simulink model "VCU_CS75_10_9_SteeringTorque"  (R2014a)
settings: Solver=FixedStepDiscrete  StartTime=0.0  StopTime=25  FixedStep=0.0005  RelTol=1e-3
undefined symbols (not defined in the file or in its folder): AutoDrivingReady, ecucoder_acal, I_SW01_L, LaterlAngleCommand, LDW, RemoteAcclPosition
libraries: simulink x880, ec5744lib x37
(part 19 of 30)

== system VCU_CS75_10_9_SteeringTorque/长安CS75底盘程序，20ms一次/Output/Subsystem/TransmitMessages10/LAS_29D/LAS_LDWShakeLevStatus ==
  LAS_LDWShakeLevStatus : Inport
  Constant{1,3..8} (7 alike) : Constant  Value=0  OutDataTypeStr=uint8
  LAS_LDWShakeLevStatusRon : Rounding  Operator=round
  LAS_LDWShakeLevStatus_1sat : Saturate  UpperLimit=48  LowerLimit=0
  LAS_LDWShakeLevStatus_Convert : DataTypeConversion  OutDataTypeStr=uint8
  LAS_LDWShakeLevStatus_Convert1 : DataTypeConversion  OutDataTypeStr=uint32
  LAS_LDWShakeLevStatus_D : Product  Inputs=*/
  LAS_LDWShakeLevStatus_F : Constant  OutDataTypeStr=single
  LAS_LDWShakeLevStatus_L : simulink/Logic and Bit Operations/Bitwise Operator  logicop=AND  UseBitMask=on  BitMask=48  BitMaskRealWorld=Stored Integer
  LAS_LDWShakeLevStatus_O : Constant  Value=0  OutDataTypeStr=single
  LAS_LDWShakeLevStatus_S : ArithShift  BitShiftNumber=-4
  LAS_LDWShakeLevStatus_sat : Saturate  UpperLimit=3  LowerLimit=0
  LAS_LDWShakeLevStatus_st : Sum  Inputs=+-
  output1 : Outport
  output2 : Outport  Port=2
  output3 : Outport  Port=3
  output4 : Outport  Port=4
  output5 : Outport  Port=5
  output6 : Outport  Port=6
  output7 : Outport  Port=7
  output8 : Outport  Port=8
  wires:
  LAS_LDWShakeLevStatus/1 -> LAS_LDWShakeLevStatus_sat/1
  LAS_LDWShakeLevStatus_sat/1 -> LAS_LDWShakeLevStatus_st/1
  LAS_LDWShakeLevStatus_O/1 -> LAS_LDWShakeLevStatus_st/2
  LAS_LDWShakeLevStatus_st/1 -> LAS_LDWShakeLevStatus_D/1
  LAS_LDWShakeLevStatus_F/1 -> LAS_LDWShakeLevStatus_D/2
  LAS_LDWShakeLevStatus_D/1 -> LAS_LDWShakeLevStatusRon/1
  LAS_LDWShakeLevStatusRon/1 -> LAS_LDWShakeLevStatus_S/1
  LAS_LDWShakeLevStatus_S/1 -> LAS_LDWShakeLevStatus_1sat/1
  LAS_LDWShakeLevStatus_1sat/1 -> LAS_LDWShakeLevStatus_Convert1/1
  LAS_LDWShakeLevStatus_Convert1/1 -> LAS_LDWShakeLevStatus_L/1
  LAS_LDWShakeLevStatus_L/1 -> LAS_LDWShakeLevStatus_Convert/1
  LAS_LDWShakeLevStatus_Convert/1 -> output2/1
  Constant1/1 -> output1/1
  Constant3/1 -> output3/1
  Constant4/1 -> output4/1
  Constant5/1 -> output5/1
  Constant6/1 -> output6/1
  Constant7/1 -> output7/1
  Constant8/1 -> output8/1

== system VCU_CS75_10_9_SteeringTorque/长安CS75底盘程序，20ms一次/Output/Subsystem/TransmitMessages10/LAS_29D/LAS_LLaneMarkerType ==
  LAS_LLaneMarkerType : Inport
  Constant{1..4,6..8} (7 alike) : Constant  Value=0  OutDataTypeStr=uint8
  LAS_LLaneMarkerTypeRon : Rounding  Operator=round
  LAS_LLaneMarkerType_1sat : Saturate  UpperLimit=7  LowerLimit=0
  LAS_LLaneMarkerType_Convert : DataTypeConversion  OutDataTypeStr=uint8
  LAS_LLaneMarkerType_Convert1 : DataTypeConversion  OutDataTypeStr=uint32
  LAS_LLaneMarkerType_D : Product  Inputs=*/
  LAS_LLaneMarkerType_F : Constant  OutDataTypeStr=single
  LAS_LLaneMarkerType_L : simulink/Logic and Bit Operations/Bitwise Operator  logicop=AND  UseBitMask=on  BitMask=7  BitMaskRealWorld=Stored Integer
  LAS_LLaneMarkerType_O : Constant  Value=0  OutDataTypeStr=single
  LAS_LLaneMarkerType_S : ArithShift
  LAS_LLaneMarkerType_sat : Saturate  UpperLimit=7  LowerLimit=0
  LAS_LLaneMarkerType_st : Sum  Inputs=+-
  output1 : Outport
  output2 : Outport  Port=2
  output3 : Outport  Port=3
  output4 : Outport  Port=4
  output5 : Outport  Port=5
  output6 : Outport  Port=6
  output7 : Outport  Port=7
  output8 : Outport  Port=8
  wires:
  LAS_LLaneMarkerType/1 -> LAS_LLaneMarkerType_sat/1
  LAS_LLaneMarkerType_sat/1 -> LAS_LLaneMarkerType_st/1
  LAS_LLaneMarkerType_O/1 -> LAS_LLaneMarkerType_st/2
  LAS_LLaneMarkerType_st/1 -> LAS_LLaneMarkerType_D/1
  LAS_LLaneMarkerType_F/1 -> LAS_LLaneMarkerType_D/2
  LAS_LLaneMarkerType_D/1 -> LAS_LLaneMarkerTypeRon/1
  LAS_LLaneMarkerTypeRon/1 -> LAS_LLaneMarkerType_S/1
  LAS_LLaneMarkerType_S/1 -> LAS_LLaneMarkerType_1sat/1
  LAS_LLaneMarkerType_1sat/1 -> LAS_LLaneMarkerType_Convert1/1
  LAS_LLaneMarkerType_Convert1/1 -> LAS_LLaneMarkerType_L/1
  LAS_LLaneMarkerType_L/1 -> LAS_LLaneMarkerType_Convert/1
  LAS_LLaneMarkerType_Convert/1 -> output5/1
  Constant1/1 -> output1/1
  Constant2/1 -> output2/1
  Constant3/1 -> output3/1
  Constant4/1 -> output4/1
  Constant6/1 -> output6/1
  Constant7/1 -> output7/1
  Constant8/1 -> output8/1

== system VCU_CS75_10_9_SteeringTorque/长安CS75底盘程序，20ms一次/Output/Subsystem/TransmitMessages10/LAS_29D/LAS_LdwSensitivityStatus ==
  LAS_LdwSensitivityStatus : Inport
  Constant{2..8} (7 alike) : Constant  Value=0  OutDataTypeStr=uint8
  LAS_LdwSensitivityStatusRon : Rounding  Operator=round
  LAS_LdwSensitivityStatus_1sat : Saturate  UpperLimit=192  LowerLimit=0
  LAS_LdwSensitivityStatus_Convert : DataTypeConversion  OutDataTypeStr=uint8
  LAS_LdwSensitivityStatus_Convert1 : DataTypeConversion  OutDataTypeStr=uint32
  LAS_LdwSensitivityStatus_D : Product  Inputs=*/
  LAS_LdwSensitivityStatus_F : Constant  OutDataTypeStr=single
  LAS_LdwSensitivityStatus_L : simulink/Logic and Bit Operations/Bitwise Operator  logicop=AND  UseBitMask=on  BitMask=192  BitMaskRealWorld=Stored Integer
  LAS_LdwSensitivityStatus_O : Constant  Value=0  OutDataTypeStr=single
  LAS_LdwSensitivityStatus_S : ArithShift  BitShiftNumber=-6
  LAS_LdwSensitivityStatus_sat : Saturate  UpperLimit=3  LowerLimit=0
  LAS_LdwSensitivityStatus_st : Sum  Inputs=+-
  output1 : Outport
  output2 : Outport  Port=2
  output3 : Outport  Port=3
  output4 : Outport  Port=4
  output5 : Outport  Port=5
  output6 : Outport  Port=6
  output7 : Outport  Port=7
  output8 : Outport  Port=8
  wires:
  LAS_LdwSensitivityStatus/1 -> LAS_LdwSensitivityStatus_sat/1
  LAS_LdwSensitivityStatus_sat/1 -> LAS_LdwSensitivityStatus_st/1
  LAS_LdwSensitivityStatus_O/1 -> LAS_LdwSensitivityStatus_st/2
  LAS_LdwSensitivityStatus_st/1 -> LAS_LdwSensitivityStatus_D/1
  LAS_LdwSensitivityStatus_F/1 -> LAS_LdwSensitivityStatus_D/2
  LAS_LdwSensitivityStatus_D/1 -> LAS_LdwSensitivityStatusRon/1
  LAS_LdwSensitivityStatusRon/1 -> LAS_LdwSensitivityStatus_S/1
  LAS_LdwSensitivityStatus_S/1 -> LAS_LdwSensitivityStatus_1sat/1
  LAS_LdwSensitivityStatus_1sat/1 -> LAS_LdwSensitivityStatus_Convert1/1
  LAS_LdwSensitivityStatus_Convert1/1 -> LAS_LdwSensitivityStatus_L/1
  LAS_LdwSensitivityStatus_L/1 -> LAS_LdwSensitivityStatus_Convert/1
  LAS_LdwSensitivityStatus_Convert/1 -> output1/1
  Constant2/1 -> output2/1
  Constant3/1 -> output3/1
  Constant4/1 -> output4/1
  Constant5/1 -> output5/1
  Constant6/1 -> output6/1
  Constant7/1 -> output7/1
  Constant8/1 -> output8/1

== system VCU_CS75_10_9_SteeringTorque/长安CS75底盘程序，20ms一次/Output/Subsystem/TransmitMessages10/LAS_29D/LAS_OverspeedSoundWarning ==
  LAS_OverspeedSoundWarning : Inport
  Constant{1..3,5..8} (7 alike) : Constant  Value=0  OutDataTypeStr=uint8
  LAS_OverspeedSoundWarningRon : Rounding  Operator=round
  LAS_OverspeedSoundWarning_1sat : Saturate  UpperLimit=192  LowerLimit=0
  LAS_OverspeedSoundWarning_Convert : DataTypeConversion  OutDataTypeStr=uint8
  LAS_OverspeedSoundWarning_Convert1 : DataTypeConversion  OutDataTypeStr=uint32
  LAS_OverspeedSoundWarning_D : Product  Inputs=*/
  LAS_OverspeedSoundWarning_F : Constant  OutDataTypeStr=single
  LAS_OverspeedSoundWarning_L : simulink/Logic and Bit Operations/Bitwise Operator  logicop=AND  UseBitMask=on  BitMask=192  BitMaskRealWorld=Stored Integer
  LAS_OverspeedSoundWarning_O : Constant  Value=0  OutDataTypeStr=single
  LAS_OverspeedSoundWarning_S : ArithShift  BitShiftNumber=-6
  LAS_OverspeedSoundWarning_sat : Saturate  UpperLimit=3  LowerLimit=0
  LAS_OverspeedSoundWarning_st : Sum  Inputs=+-
  output1 : Outport
  output2 : Outport  Port=2
  output3 : Outport  Port=3
  output4 : Outport  Port=4
  output5 : Outport  Port=5
  output6 : Outport  Port=6
  output7 : Outport  Port=7
  output8 : Outport  Port=8
  wires:
  LAS_OverspeedSoundWarning/1 -> LAS_OverspeedSoundWarning_sat/1
  LAS_OverspeedSoundWarning_sat/1 -> LAS_OverspeedSoundWarning_st/1
  LAS_OverspeedSoundWarning_O/1 -> LAS_OverspeedSoundWarning_st/2
  LAS_OverspeedSoundWarning_st/1 -> LAS_OverspeedSoundWarning_D/1
  LAS_OverspeedSoundWarning_F/1 -> LAS_OverspeedSoundWarning_D/2
  LAS_OverspeedSoundWarning_D/1 -> LAS_OverspeedSoundWarningRon/1
  LAS_OverspeedSoundWarningRon/1 -> LAS_OverspeedSoundWarning_S/1
  LAS_OverspeedSoundWarning_S/1 -> LAS_OverspeedSoundWarning_1sat/1
  LAS_OverspeedSoundWarning_1sat/1 -> LAS_OverspeedSoundWarning_Convert1/1
  LAS_OverspeedSoundWarning_Convert1/1 -> LAS_OverspeedSoundWarning_L/1
  LAS_OverspeedSoundWarning_L/1 -> LAS_OverspeedSoundWarning_Convert/1
  LAS_OverspeedSoundWarning_Convert/1 -> output4/1
  Constant1/1 -> output1/1
  Constant2/1 -> output2/1
  Constant3/1 -> output3/1
  Constant5/1 -> output5/1
  Constant6/1 -> output6/1
  Constant7/1 -> output7/1
  Constant8/1 -> output8/1

== system VCU_CS75_10_9_SteeringTorque/长安CS75底盘程序，20ms一次/Output/Subsystem/TransmitMessages10/LAS_29D/LAS_OverspeedSoundWarningEnSt ==
  LAS_OverspeedSoundWarningEnSt : Inport
  Constant{1,3..8} (7 alike) : Constant  Value=0  OutDataTypeStr=uint8
  LAS_OverspeedSoundWarningEnStRon : Rounding  Operator=round
  LAS_OverspeedSoundWarningEnSt_1sat : Saturate  UpperLimit=3  LowerLimit=0
  LAS_OverspeedSoundWarningEnSt_Convert : DataTypeConversion  OutDataTypeStr=uint8
  LAS_OverspeedSoundWarningEnSt_Convert1 : DataTypeConversion  OutDataTypeStr=uint32
  LAS_OverspeedSoundWarningEnSt_D : Product  Inputs=*/
  LAS_OverspeedSoundWarningEnSt_F : Constant  OutDataTypeStr=single
  LAS_OverspeedSoundWarningEnSt_L : simulink/Logic and Bit Operations/Bitwise Operator  logicop=AND  UseBitMask=on  BitMask=3  BitMaskRealWorld=Stored Integer
  LAS_OverspeedSoundWarningEnSt_O : Constant  Value=0  OutDataTypeStr=single
  LAS_OverspeedSoundWarningEnSt_S : ArithShift
  LAS_OverspeedSoundWarningEnSt_sat : Saturate  UpperLimit=3  LowerLimit=0
  LAS_OverspeedSoundWarningEnSt_st : Sum  Inputs=+-
  output1 : Outport
  output2 : Outport  Port=2
  output3 : Outport  Port=3
  output4 : Outport  Port=4
  output5 : Outport  Port=5
  output6 : Outport  Port=6
  output7 : Outport  Port=7
  output8 : Outport  Port=8
  wires:
  LAS_OverspeedSoundWarningEnSt/1 -> LAS_OverspeedSoundWarningEnSt_sat/1
  LAS_OverspeedSoundWarningEnSt_sat/1 -> LAS_OverspeedSoundWarningEnSt_st/1
  LAS_OverspeedSoundWarningEnSt_O/1 -> LAS_OverspeedSoundWarningEnSt_st/2
  LAS_OverspeedSoundWarningEnSt_st/1 -> LAS_OverspeedSoundWarningEnSt_D/1
  LAS_OverspeedSoundWarningEnSt_F/1 -> LAS_OverspeedSoundWarningEnSt_D/2
  LAS_OverspeedSoundWarningEnSt_D/1 -> LAS_OverspeedSoundWarningEnStRon/1
  LAS_OverspeedSoundWarningEnStRon/1 -> LAS_OverspeedSoundWarningEnSt_S/1
  LAS_OverspeedSoundWarningEnSt_S/1 -> LAS_OverspeedSoundWarningEnSt_1sat/1
  LAS_OverspeedSoundWarningEnSt_1sat/1 -> LAS_OverspeedSoundWarningEnSt_Convert1/1
  LAS_OverspeedSoundWarningEnSt_Convert1/1 -> LAS_OverspeedSoundWarningEnSt_L/1
  LAS_OverspeedSoundWarningEnSt_L/1 -> LAS_OverspeedSoundWarningEnSt_Convert/1
  LAS_OverspeedSoundWarningEnSt_Convert/1 -> output2/1
  Constant1/1 -> output1/1
  Constant3/1 -> output3/1
  Constant4/1 -> output4/1
  Constant5/1 -> output5/1
  Constant6/1 -> output6/1
  Constant7/1 -> output7/1
  Constant8/1 -> output8/1

== system VCU_CS75_10_9_SteeringTorque/长安CS75底盘程序，20ms一次/Output/Subsystem/TransmitMessages10/LAS_29D/LAS_OverspeedVisualWarning ==
  LAS_OverspeedVisualWarning : Inport
  Constant{1..4,6..8} (7 alike) : Constant  Value=0  OutDataTypeStr=uint8
  LAS_OverspeedVisualWarningRon : Rounding  Operator=round
  LAS_OverspeedVisualWarning_1sat : Saturate  UpperLimit=192  LowerLimit=0
  LAS_OverspeedVisualWarning_Convert : DataTypeConversion  OutDataTypeStr=uint8
  LAS_OverspeedVisualWarning_Convert1 : DataTypeConversion  OutDataTypeStr=uint32
  LAS_OverspeedVisualWarning_D : Product  Inputs=*/
  LAS_OverspeedVisualWarning_F : Constant  OutDataTypeStr=single
  LAS_OverspeedVisualWarning_L : simulink/Logic and Bit Operations/Bitwise Operator  logicop=AND  UseBitMask=on  BitMask=192  BitMaskRealWorld=Stored Integer
  LAS_OverspeedVisualWarning_O : Constant  Value=0  OutDataTypeStr=single
  LAS_OverspeedVisualWarning_S : ArithShift  BitShiftNumber=-6
  LAS_OverspeedVisualWarning_sat : Saturate  UpperLimit=3  LowerLimit=0
  LAS_OverspeedVisualWarning_st : Sum  Inputs=+-
  output1 : Outport
  output2 : Outport  Port=2
  output3 : Outport  Port=3
  output4 : Outport  Port=4
  output5 : Outport  Port=5
  output6 : Outport  Port=6
  output7 : Outport  Port=7
  output8 : Outport  Port=8
  wires:
  LAS_OverspeedVisualWarning/1 -> LAS_OverspeedVisualWarning_sat/1
  LAS_OverspeedVisualWarning_sat/1 -> LAS_OverspeedVisualWarning_st/1
  LAS_OverspeedVisualWarning_O/1 -> LAS_OverspeedVisualWarning_st/2
  LAS_OverspeedVisualWarning_st/1 -> LAS_OverspeedVisualWarning_D/1
  LAS_OverspeedVisualWarning_F/1 -> LAS_OverspeedVisualWarning_D/2
  LAS_OverspeedVisualWarning_D/1 -> LAS_OverspeedVisualWarningRon/1
  LAS_OverspeedVisualWarningRon/1 -> LAS_OverspeedVisualWarning_S/1
  LAS_OverspeedVisualWarning_S/1 -> LAS_OverspeedVisualWarning_1sat/1
  LAS_OverspeedVisualWarning_1sat/1 -> LAS_OverspeedVisualWarning_Convert1/1
  LAS_OverspeedVisualWarning_Convert1/1 -> LAS_OverspeedVisualWarning_L/1
  LAS_OverspeedVisualWarning_L/1 -> LAS_OverspeedVisualWarning_Convert/1
  LAS_OverspeedVisualWarning_Convert/1 -> output5/1
  Constant1/1 -> output1/1
  Constant2/1 -> output2/1
  Constant3/1 -> output3/1
  Constant4/1 -> output4/1
  Constant6/1 -> output6/1
  Constant7/1 -> output7/1
  Constant8/1 -> output8/1

== system VCU_CS75_10_9_SteeringTorque/长安CS75底盘程序，20ms一次/Output/Subsystem/TransmitMessages10/LAS_29D/LAS_OverspeedWarningEnableStatus ==
  LAS_OverspeedWarningEnableStatus : Inport
  Constant{1..3,5..8} (7 alike) : Constant  Value=0  OutDataTypeStr=uint8
  LAS_OverspeedWarningEnableStatusRon : Rounding  Operator=round
  LAS_OverspeedWarningEnableStatus_1sat : Saturate  UpperLimit=48  LowerLimit=0
  LAS_OverspeedWarningEnableStatus_Convert : DataTypeConversion  OutDataTypeStr=uint8
  LAS_OverspeedWarningEnableStatus_Convert1 : DataTypeConversion  OutDataTypeStr=uint32
  LAS_OverspeedWarningEnableStatus_D : Product  Inputs=*/
  LAS_OverspeedWarningEnableStatus_F : Constant  OutDataTypeStr=single
  LAS_OverspeedWarningEnableStatus_L : simulink/Logic and Bit Operations/Bitwise Operator  logicop=AND  UseBitMask=on  BitMask=48  BitMaskRealWorld=Stored Integer
  LAS_OverspeedWarningEnableStatus_O : Constant  Value=0  OutDataTypeStr=single
  LAS_OverspeedWarningEnableStatus_S : ArithShift  BitShiftNumber=-4
  LAS_OverspeedWarningEnableStatus_sat : Saturate  UpperLimit=3  LowerLimit=0
  LAS_OverspeedWarningEnableStatus_st : Sum  Inputs=+-
  output1 : Outport
  output2 : Outport  Port=2
  output3 : Outport  Port=3
  output4 : Outport  Port=4
  output5 : Outport  Port=5
  output6 : Outport  Port=6
  output7 : Outport  Port=7
  output8 : Outport  Port=8
  wires:
  LAS_OverspeedWarningEnableStatus/1 -> LAS_OverspeedWarningEnableStatus_sat/1
  LAS_OverspeedWarningEnableStatus_sat/1 -> LAS_OverspeedWarningEnableStatus_st/1
  LAS_OverspeedWarningEnableStatus_O/1 -> LAS_OverspeedWarningEnableStatus_st/2
  LAS_OverspeedWarningEnableStatus_st/1 -> LAS_OverspeedWarningEnableStatus_D/1
  LAS_OverspeedWarningEnableStatus_F/1 -> LAS_OverspeedWarningEnableStatus_D/2
  LAS_OverspeedWarningEnableStatus_D/1 -> LAS_OverspeedWarningEnableStatusRon/1
  LAS_OverspeedWarningEnableStatusRon/1 -> LAS_OverspeedWarningEnableStatus_S/1
  LAS_OverspeedWarningEnableStatus_S/1 -> LAS_OverspeedWarningEnableStatus_1sat/1
  LAS_OverspeedWarningEnableStatus_1sat/1 -> LAS_OverspeedWarningEnableStatus_Convert1/1
  LAS_OverspeedWarningEnableStatus_Convert1/1 -> LAS_OverspeedWarningEnableStatus_L/1
  LAS_OverspeedWarningEnableStatus_L/1 -> LAS_OverspeedWarningEnableStatus_Convert/1
  LAS_OverspeedWarningEnableStatus_Convert/1 -> output4/1
  Constant1/1 -> output1/1
  Constant2/1 -> output2/1
  Constant3/1 -> output3/1
  Constant5/1 -> output5/1
  Constant6/1 -> output6/1
  Constant7/1 -> output7/1
  Constant8/1 -> output8/1

== system VCU_CS75_10_9_SteeringTorque/长安CS75底盘程序，20ms一次/Output/Subsystem/TransmitMessages10/LAS_29D/LAS_OverspeedWarningOffset ==
  LAS_OverspeedWarningOffset : Inport
  Constant{1..5,7..8} (7 alike) : Constant  Value=0  OutDataTypeStr=uint8
  LAS_OverspeedWarningOffsetRon : Rounding  Operator=round
  LAS_OverspeedWarningOffset_1sat : Saturate  UpperLimit=248  LowerLimit=0
  LAS_OverspeedWarningOffset_Convert : DataTypeConversion  OutDataTypeStr=uint8
  LAS_OverspeedWarningOffset_Convert1 : DataTypeConversion  OutDataTypeStr=uint32
  LAS_OverspeedWarningOffset_D : Product  Inputs=*/
  LAS_OverspeedWarningOffset_F : Constant  OutDataTypeStr=single
  LAS_OverspeedWarningOffset_L : simulink/Logic and Bit Operations/Bitwise Operator  logicop=AND  UseBitMask=on  BitMask=248  BitMaskRealWorld=Stored Integer
  LAS_OverspeedWarningOffset_O : Constant  Value=-10  OutDataTypeStr=single
  LAS_OverspeedWarningOffset_S : ArithShift  BitShiftNumber=-3
  LAS_OverspeedWarningOffset_sat : Saturate  UpperLimit=10  LowerLimit=-10
  LAS_OverspeedWarningOffset_st : Sum  Inputs=+-
  output1 : Outport
  output2 : Outport  Port=2
  output3 : Outport  Port=3
  output4 : Outport  Port=4
  output5 : Outport  Port=5
  output6 : Outport  Port=6
  output7 : Outport  Port=7
  output8 : Outport  Port=8
  wires:
  LAS_OverspeedWarningOffset/1 -> LAS_OverspeedWarningOffset_sat/1
  LAS_OverspeedWarningOffset_sat/1 -> LAS_OverspeedWarningOffset_st/1
  LAS_OverspeedWarningOffset_O/1 -> LAS_OverspeedWarningOffset_st/2
  LAS_OverspeedWarningOffset_st/1 -> LAS_OverspeedWarningOffset_D/1
  LAS_OverspeedWarningOffset_F/1 -> LAS_OverspeedWarningOffset_D/2
  LAS_OverspeedWarningOffset_D/1 -> LAS_OverspeedWarningOffsetRon/1
  LAS_OverspeedWarningOffsetRon/1 -> LAS_OverspeedWarningOffset_S/1
  LAS_OverspeedWarningOffset_S/1 -> LAS_OverspeedWarningOffset_1sat/1
  LAS_OverspeedWarningOffset_1sat/1 -> LAS_OverspeedWarningOffset_Convert1/1
  LAS_OverspeedWarningOffset_Convert1/1 -> LAS_OverspeedWarningOffset_L/1
  LAS_OverspeedWarningOffset_L/1 -> LAS_OverspeedWarningOffset_Convert/1
  LAS_OverspeedWarningOffset_Convert/1 -> output6/1
  Constant1/1 -> output1/1
  Constant2/1 -> output2/1
  Constant3/1 -> output3/1
  Constant4/1 -> output4/1
  Constant5/1 -> output5/1
  Constant7/1 -> output7/1
  Constant8/1 -> output8/1

== system VCU_CS75_10_9_SteeringTorque/长安CS75底盘程序，20ms一次/Output/Subsystem/TransmitMessages10/LAS_29D/LAS_RLaneMarkerType ==
  LAS_RLaneMarkerType : Inport
  Constant{1..5,7..8} (7 alike) : Constant  Value=0  OutDataTypeStr=uint8
  LAS_RLaneMarkerTypeRon : Rounding  Operator=round
  LAS_RLaneMarkerType_1sat : Saturate  UpperLimit=7  LowerLimit=0
  LAS_RLaneMarkerType_Convert : DataTypeConversion  OutDataTypeStr=uint8
  LAS_RLaneMarkerType_Convert1 : DataTypeConversion  OutDataTypeStr=uint32
  LAS_RLaneMarkerType_D : Product  Inputs=*/
  LAS_RLaneMarkerType_F : Constant  OutDataTypeStr=single
  LAS_RLaneMarkerType_L : simulink/Logic and Bit Operations/Bitwise Operator  logicop=AND  UseBitMask=on  BitMask=7  BitMaskRealWorld=Stored Integer
  LAS_RLaneMarkerType_O : Constant  Value=0  OutDataTypeStr=single
  LAS_RLaneMarkerType_S : ArithShift
  LAS_RLaneMarkerType_sat : Saturate  UpperLimit=7  LowerLimit=0
  LAS_RLaneMarkerType_st : Sum  Inputs=+-
  output1 : Outport
  output2 : Outport  Port=2
  output3 : Outport  Port=3
  output4 : Outport  Port=4
  output5 : Outport  Port=5
  output6 : Outport  Port=6
  output7 : Outport  Port=7
  output8 : Outport  Port=8
  wires:
  LAS_RLaneMarkerType/1 -> LAS_RLaneMarkerType_sat/1
  LAS_RLaneMarkerType_sat/1 -> LAS_RLaneMarkerType_st/1
  LAS_RLaneMarkerType_O/1 -> LAS_RLaneMarkerType_st/2
  LAS_RLaneMarkerType_st/1 -> LAS_RLaneMarkerType_D/1
  LAS_RLaneMarkerType_F/1 -> LAS_RLaneMarkerType_D/2
  LAS_RLaneMarkerType_D/1 -> LAS_RLaneMarkerTypeRon/1
  LAS_RLaneMarkerTypeRon/1 -> LAS_RLaneMarkerType_S/1
  LAS_RLaneMarkerType_S/1 -> LAS_RLaneMarkerType_1sat/1
  LAS_RLaneMarkerType_1sat/1 -> LAS_RLaneMarkerType_Convert1/1
  LAS_RLaneMarkerType_Convert1/1 -> LAS_RLaneMarkerType_L/1
  LAS_RLaneMarkerType_L/1 -> LAS_RLaneMarkerType_Convert/1
  LAS_RLaneMarkerType_Convert/1 -> output6/1
  Constant1/1 -> output1/1
  Constant2/1 -> output2/1
  Constant3/1 -> output3/1
  Constant4/1 -> output4/1
  Constant5/1 -> output5/1
  Constant7/1 -> output7/1
  Constant8/1 -> output8/1

== system VCU_CS75_10_9_SteeringTorque/长安CS75底盘程序，20ms一次/Output/Subsystem/TransmitMessages10/LAS_29D/LAS_SLASwitchStatus ==
  LAS_SLASwitchStatus : Inport
  Constant{2..8} (7 alike) : Constant  Value=0  OutDataTypeStr=uint8
  LAS_SLASwitchStatusRon : Rounding  Operator=round
  LAS_SLASwitchStatus_1sat : Saturate  UpperLimit=2  LowerLimit=0
  LAS_SLASwitchStatus_Convert : DataTypeConversion  OutDataTypeStr=uint8
  LAS_SLASwitchStatus_Convert1 : DataTypeConversion  OutDataTypeStr=uint32
  LAS_SLASwitchStatus_D : Product  Inputs=*/
  LAS_SLASwitchStatus_F : Constant  OutDataTypeStr=single
  LAS_SLASwitchStatus_L : simulink/Logic and Bit Operations/Bitwise Operator  logicop=AND  UseBitMask=on  BitMask=2  BitMaskRealWorld=Stored Integer
  LAS_SLASwitchStatus_O : Constant  Value=0  OutDataTypeStr=single
  LAS_SLASwitchStatus_S : ArithShift  BitShiftNumber=-1
  LAS_SLASwitchStatus_sat : Saturate  UpperLimit=1  LowerLimit=0
  LAS_SLASwitchStatus_st : Sum  Inputs=+-
  output1 : Outport
  output2 : Outport  Port=2
  output3 : Outport  Port=3
  output4 : Outport  Port=4
  output5 : Outport  Port=5
  output6 : Outport  Port=6
  output7 : Outport  Port=7
  output8 : Outport  Port=8
  wires:
  LAS_SLASwitchStatus/1 -> LAS_SLASwitchStatus_sat/1
  LAS_SLASwitchStatus_sat/1 -> LAS_SLASwitchStatus_st/1
  LAS_SLASwitchStatus_O/1 -> LAS_SLASwitchStatus_st/2
  LAS_SLASwitchStatus_st/1 -> LAS_SLASwitchStatus_D/1
  LAS_SLASwitchStatus_F/1 -> LAS_SLASwitchStatus_D/2
  LAS_SLASwitchStatus_D/1 -> LAS_SLASwitchStatusRon/1
  LAS_SLASwitchStatusRon/1 -> LAS_SLASwitchStatus_S/1
  LAS_SLASwitchStatus_S/1 -> LAS_SLASwitchStatus_1sat/1
  LAS_SLASwitchStatus_1sat/1 -> LAS_SLASwitchStatus_Convert1/1
  LAS_SLASwitchStatus_Convert1/1 -> LAS_SLASwitchStatus_L/1
  LAS_SLASwitchStatus_L/1 -> LAS_SLASwitchStatus_Convert/1
  LAS_SLASwitchStatus_Convert/1 -> output1/1
  Constant2/1 -> output2/1
  Constant3/1 -> output3/1
  Constant4/1 -> output4/1
  Constant5/1 -> output5/1
  Constant6/1 -> output6/1
  Constant7/1 -> output7/1
  Constant8/1 -> output8/1

== system VCU_CS75_10_9_SteeringTorque/长安CS75底盘程序，20ms一次/Output/Subsystem/TransmitMessages10/LAS_29D/LAS_VoiceWarning ==
  LAS_VoiceWarning : Inport
  Constant{1..2,4..8} (7 alike) : Constant  Value=0  OutDataTypeStr=uint8
  LAS_VoiceWarningRon : Rounding  Operator=round
  LAS_VoiceWarning_1sat : Saturate  UpperLimit=192  LowerLimit=0
  LAS_VoiceWarning_Convert : DataTypeConversion  OutDataTypeStr=uint8
  LAS_VoiceWarning_Convert1 : DataTypeConversion  OutDataTypeStr=uint32
  LAS_VoiceWarning_D : Product  Inputs=*/
  LAS_VoiceWarning_F : Constant  OutDataTypeStr=single
  LAS_VoiceWarning_L : simulink/Logic and Bit Operations/Bitwise Operator  logicop=AND  UseBitMask=on  BitMask=192  BitMaskRealWorld=Stored Integer
  LAS_VoiceWarning_O : Constant  Value=0  OutDataTypeStr=single
  LAS_VoiceWarning_S : ArithShift  BitShiftNumber=-6
  LAS_VoiceWarning_sat : Saturate  UpperLimit=0  LowerLimit=0
  LAS_VoiceWarning_st : Sum  Inputs=+-
  output1 : Outport
  output2 : Outport  Port=2
  output3 : Outport  Port=3
  output4 : Outport  Port=4
  output5 : Outport  Port=5
  output6 : Outport  Port=6
  output7 : Outport  Port=7
  output8 : Outport  Port=8
  wires:
  LAS_VoiceWarning/1 -> LAS_VoiceWarning_sat/1
  LAS_VoiceWarning_sat/1 -> LAS_VoiceWarning_st/1
  LAS_VoiceWarning_O/1 -> LAS_VoiceWarning_st/2
  LAS_VoiceWarning_st/1 -> LAS_VoiceWarning_D/1
  LAS_VoiceWarning_F/1 -> LAS_VoiceWarning_D/2
  LAS_VoiceWarning_D/1 -> LAS_VoiceWarningRon/1
  LAS_VoiceWarningRon/1 -> LAS_VoiceWarning_S/1
  LAS_VoiceWarning_S/1 -> LAS_VoiceWarning_1sat/1
  LAS_VoiceWarning_1sat/1 -> LAS_VoiceWarning_Convert1/1
  LAS_VoiceWarning_Convert1/1 -> LAS_VoiceWarning_L/1
  LAS_VoiceWarning_L/1 -> LAS_VoiceWarning_Convert/1
  LAS_VoiceWarning_Convert/1 -> output3/1
  Constant1/1 -> output1/1
  Constant2/1 -> output2/1
  Constant4/1 -> output4/1
  Constant5/1 -> output5/1
  Constant6/1 -> output6/1
  Constant7/1 -> output7/1
  Constant8/1 -> output8/1

== system VCU_CS75_10_9_SteeringTorque/长安CS75底盘程序，20ms一次/Output/Subsystem/TransmitMessages10/LAS_29D/RollingConter ==
  RollingConter : Inport
  Constant{1..6,8} (7 alike) : Constant  Value=0  OutDataTypeStr=uint8
  RollingConterRon : Rounding  Operator=round
  RollingConter_1sat : Saturate  UpperLimit=15  LowerLimit=0
  RollingConter_Convert : DataTypeConversion  OutDataTypeStr=uint8
  RollingConter_Convert1 : DataTypeConversion  OutDataTypeStr=uint32
  RollingConter_D : Product  Inputs=*/
  RollingConter_F : Constant  OutDataTypeStr=single
  RollingConter_L : simulink/Logic and Bit Operations/Bitwise Operator  logicop=AND  UseBitMask=on  BitMask=15  BitMaskRealWorld=Stored Integer
  RollingConter_O : Constant  Value=0  OutDataTypeStr=single
  RollingConter_S : ArithShift
  RollingConter_sat : Saturate  UpperLimit=0  LowerLimit=0
  RollingConter_st : Sum  Inputs=+-
  output1 : Outport
  output2 : Outport  Port=2
  output3 : Outport  Port=3
  output4 : Outport  Port=4
  output5 : Outport  Port=5
  output6 : Outport  Port=6
  output7 : Outport  Port=7
  output8 : Outport  Port=8
  wires:
  RollingConter/1 -> RollingConter_sat/1
  RollingConter_sat/1 -> RollingConter_st/1
  RollingConter_O/1 -> RollingConter_st/2
  RollingConter_st/1 -> RollingConter_D/1
  RollingConter_F/1 -> RollingConter_D/2
  RollingConter_D/1 -> RollingConterRon/1
  RollingConterRon/1 -> RollingConter_S/1
  RollingConter_S/1 -> RollingConter_1sat/1
  RollingConter_1sat/1 -> RollingConter_Convert1/1
  RollingConter_Convert1/1 -> RollingConter_L/1
  RollingConter_L/1 -> RollingConter_Convert/1
  RollingConter_Convert/1 -> output7/1
  Constant1/1 -> output1/1
  Constant2/1 -> output2/1
  Constant3/1 -> output3/1
  Constant4/1 -> output4/1
  Constant5/1 -> output5/1
  Constant6/1 -> output6/1
  Constant8/1 -> output8/1

== system VCU_CS75_10_9_SteeringTorque/长安CS75底盘程序，20ms一次/Output/Subsystem/TransmitMessages11/GW_LCDAL_2EA/LCDAL_AudioWarningEnableStatus ==
  LCDAL_AudioWarningEnableStatus : Inport
  Constant{1..4,6..8} (7 alike) : Constant  Value=0  OutDataTypeStr=uint8
  LCDAL_AudioWarningEnableStatusABS : Abs
  LCDAL_AudioWarningEnableStatusCS : ArithShift  BitShiftNumber=-2
  LCDAL_AudioWarningEnableStatusConS : Constant  OutDataTypeStr=single
  LCDAL_AudioWarningEnableStatusCosR : Constant  Value=0  OutDataTypeStr=uint8
  LCDAL_AudioWarningEnableStatusROP : RelationalOperator  Operator=<  OutDataTypeStr=boolean
  LCDAL_AudioWarningEnableStatusRon : Rounding  Operator=round
  LCDAL_AudioWarningEnableStatusSW : Switch  Criteria=u2 ~= 0
  LCDAL_AudioWarningEnableStatus_1sat : Saturate  UpperLimit=192  LowerLimit=0
  LCDAL_AudioWarningEnableStatus_Convert : DataTypeConversion  OutDataTypeStr=uint8
  LCDAL_AudioWarningEnableStatus_Convert1 : DataTypeConversion  OutDataTypeStr=uint32
  LCDAL_AudioWarningEnableStatus_D : Product  Inputs=*/
  LCDAL_AudioWarningEnableStatus_F : Constant  OutDataTypeStr=single
  LCDAL_AudioWarningEnableStatus_L : simulink/Logic and Bit Operations/Bitwise Operator  logicop=AND  UseBitMask=on  BitMask=192  BitMaskRealWorld=Stored Integer
  LCDAL_AudioWarningEnableStatus_O : Constant  Value=0  OutDataTypeStr=single
  LCDAL_AudioWarningEnableStatus_S : ArithShift  BitShiftNumber=-6
  LCDAL_AudioWarningEnableStatus_sat : Saturate  UpperLimit=3  LowerLimit=0
  LCDAL_AudioWarningEnableStatus_st : Sum  Inputs=+-
  LCDAL_AudioWarningEnableStatussubcon : Sum  Inputs=+-
  output1 : Outport
  output2 : Outport  Port=2
  output3 : Outport  Port=3
  output4 : Outport  Port=4
  output5 : Outport  Port=5
  output6 : Outport  Port=6
  output7 : Outport  Port=7
  output8 : Outport  Port=8
  wires:
  Constant8/1 -> output8/1
  Constant7/1 -> output7/1
  Constant6/1 -> output6/1
  Constant4/1 -> output4/1
  Constant3/1 -> output3/1
  Constant2/1 -> output2/1
  Constant1/1 -> output1/1
  LCDAL_AudioWarningEnableStatus_Convert/1 -> output5/1
  LCDAL_AudioWarningEnableStatus_L/1 -> LCDAL_AudioWarningEnableStatus_Convert/1
  LCDAL_AudioWarningEnableStatus_Convert1/1 -> LCDAL_AudioWarningEnableStatus_L/1
  LCDAL_AudioWarningEnableStatus_1sat/1 -> LCDAL_AudioWarningEnableStatus_Convert1/1
  LCDAL_AudioWarningEnableStatus_S/1 -> LCDAL_AudioWarningEnableStatus_1sat/1
  LCDAL_AudioWarningEnableStatusSW/1 -> LCDAL_AudioWarningEnableStatus_S/1
  LCDAL_AudioWarningEnableStatusROP/1 -> LCDAL_AudioWarningEnableStatusSW/2
  LCDAL_AudioWarningEnableStatussubcon/1 -> LCDAL_AudioWarningEnableStatusSW/1
  LCDAL_AudioWarningEnableStatusABS/1 -> LCDAL_AudioWarningEnableStatussubcon/2
  LCDAL_AudioWarningEnableStatusCS/1 -> LCDAL_AudioWarningEnableStatussubcon/1
  LCDAL_AudioWarningEnableStatusConS/1 -> LCDAL_AudioWarningEnableStatusCS/1
  LCDAL_AudioWarningEnableStatusCosR/1 -> LCDAL_AudioWarningEnableStatusROP/2
  LCDAL_AudioWarningEnableStatusRon/1 -> LCDAL_AudioWarningEnableStatusSW/3, LCDAL_AudioWarningEnableStatusABS/1, LCDAL_AudioWarningEnableStatusROP/1
  LCDAL_AudioWarningEnableStatus_D/1 -> LCDAL_AudioWarningEnableStatusRon/1
  LCDAL_AudioWarningEnableStatus_F/1 -> LCDAL_AudioWarningEnableStatus_D/2
  LCDAL_AudioWarningEnableStatus_st/1 -> LCDAL_AudioWarningEnableStatus_D/1
  LCDAL_AudioWarningEnableStatus_O/1 -> LCDAL_AudioWarningEnableStatus_st/2
  LCDAL_AudioWarningEnableStatus_sat/1 -> LCDAL_AudioWarningEnableStatus_st/1
  LCDAL_AudioWarningEnableStatus/1 -> LCDAL_AudioWarningEnableStatus_sat/1

== system VCU_CS75_10_9_SteeringTorque/长安CS75底盘程序，20ms一次/Output/Subsystem/TransmitMessages11/GW_LCDAL_2EA/LCDAL_BSDLCAAlert ==
  LCDAL_BSDLCAAlert : Inport
  Constant{2..8} (7 alike) : Constant  Value=0  OutDataTypeStr=uint8
  LCDAL_BSDLCAAlertRon : Rounding  Operator=round
  LCDAL_BSDLCAAlert_1sat : Saturate  UpperLimit=48  LowerLimit=0
  LCDAL_BSDLCAAlert_Convert : DataTypeConversion  OutDataTypeStr=uint8
  LCDAL_BSDLCAAlert_Convert1 : DataTypeConversion  OutDataTypeStr=uint32
  LCDAL_BSDLCAAlert_D : Product  Inputs=*/
  LCDAL_BSDLCAAlert_F : Constant  OutDataTypeStr=single
  LCDAL_BSDLCAAlert_L : simulink/Logic and Bit Operations/Bitwise Operator  logicop=AND  UseBitMask=on  BitMask=48  BitMaskRealWorld=Stored Integer
  LCDAL_BSDLCAAlert_O : Constant  Value=0  OutDataTypeStr=single
  LCDAL_BSDLCAAlert_S : ArithShift  BitShiftNumber=-4
  LCDAL_BSDLCAAlert_sat : Saturate  UpperLimit=3  LowerLimit=0
  LCDAL_BSDLCAAlert_st : Sum  Inputs=+-
  output1 : Outport
  output2 : Outport  Port=2
  output3 : Outport  Port=3
  output4 : Outport  Port=4
  output5 : Outport  Port=5
  output6 : Outport  Port=6
  output7 : Outport  Port=7
  output8 : Outport  Port=8
  wires:
  Constant8/1 -> output8/1
  Constant7/1 -> output7/1
  Constant6/1 -> output6/1
  Constant5/1 -> output5/1
  Constant4/1 -> output4/1
  Constant3/1 -> output3/1
  Constant2/1 -> output2/1
  LCDAL_BSDLCAAlert_Convert/1 -> output1/1
  LCDAL_BSDLCAAlert_L/1 -> LCDAL_BSDLCAAlert_Convert/1
  LCDAL_BSDLCAAlert_Convert1/1 -> LCDAL_BSDLCAAlert_L/1
  LCDAL_BSDLCAAlert_1sat/1 -> LCDAL_BSDLCAAlert_Convert1/1
  LCDAL_BSDLCAAlert_S/1 -> LCDAL_BSDLCAAlert_1sat/1
  LCDAL_BSDLCAAlertRon/1 -> LCDAL_BSDLCAAlert_S/1
  LCDAL_BSDLCAAlert_D/1 -> LCDAL_BSDLCAAlertRon/1
  LCDAL_BSDLCAAlert_F/1 -> LCDAL_BSDLCAAlert_D/2
  LCDAL_BSDLCAAlert_st/1 -> LCDAL_BSDLCAAlert_D/1
  LCDAL_BSDLCAAlert_O/1 -> LCDAL_BSDLCAAlert_st/2
  LCDAL_BSDLCAAlert_sat/1 -> LCDAL_BSDLCAAlert_st/1
  LCDAL_BSDLCAAlert/1 -> LCDAL_BSDLCAAlert_sat/1

== system VCU_CS75_10_9_SteeringTorque/长安CS75底盘程序，20ms一次/Output/Subsystem/TransmitMessages11/GW_LCDAL_2EA/LCDAL_BSDLCAEnableStatus ==
  LCDAL_BSDLCAEnableStatus : Inport
  Constant{2..8} (7 alike) : Constant  Value=0  OutDataTypeStr=uint8
  LCDAL_BSDLCAEnableStatusRon : Rounding  Operator=round
  LCDAL_BSDLCAEnableStatus_1sat : Saturate  UpperLimit=192  LowerLimit=0
  LCDAL_BSDLCAEnableStatus_Convert : DataTypeConversion  OutDataTypeStr=uint8
  LCDAL_BSDLCAEnableStatus_Convert1 : DataTypeConversion  OutDataTypeStr=uint32
  LCDAL_BSDLCAEnableStatus_D : Product  Inputs=*/
  LCDAL_BSDLCAEnableStatus_F : Constant  OutDataTypeStr=single
  LCDAL_BSDLCAEnableStatus_L : simulink/Logic and Bit Operations/Bitwise Operator  logicop=AND  UseBitMask=on  BitMask=192  BitMaskRealWorld=Stored Integer
  LCDAL_BSDLCAEnableStatus_O : Constant  Value=0  OutDataTypeStr=single
  LCDAL_BSDLCAEnableStatus_S : ArithShift  BitShiftNumber=-6
  LCDAL_BSDLCAEnableStatus_sat : Saturate  UpperLimit=3  LowerLimit=0
  LCDAL_BSDLCAEnableStatus_st : Sum  Inputs=+-
  output1 : Outport
  output2 : Outport  Port=2
  output3 : Outport  Port=3
  output4 : Outport  Port=4
  output5 : Outport  Port=5
  output6 : Outport  Port=6
  output7 : Outport  Port=7
  output8 : Outport  Port=8
  wires:
  Constant8/1 -> output8/1
  Constant7/1 -> output7/1
  Constant6/1 -> output6/1
  Constant5/1 -> output5/1
  Constant4/1 -> output4/1
  Constant3/1 -> output3/1
  Constant2/1 -> output2/1
  LCDAL_BSDLCAEnableStatus_Convert/1 -> output1/1
  LCDAL_BSDLCAEnableStatus_L/1 -> LCDAL_BSDLCAEnableStatus_Convert/1
  LCDAL_BSDLCAEnableStatus_Convert1/1 -> LCDAL_BSDLCAEnableStatus_L/1
  LCDAL_BSDLCAEnableStatus_1sat/1 -> LCDAL_BSDLCAEnableStatus_Convert1/1
  LCDAL_BSDLCAEnableStatus_S/1 -> LCDAL_BSDLCAEnableStatus_1sat/1
  LCDAL_BSDLCAEnableStatusRon/1 -> LCDAL_BSDLCAEnableStatus_S/1
  LCDAL_BSDLCAEnableStatus_D/1 -> LCDAL_BSDLCAEnableStatusRon/1
  LCDAL_BSDLCAEnableStatus_F/1 -> LCDAL_BSDLCAEnableStatus_D/2
  LCDAL_BSDLCAEnableStatus_st/1 -> LCDAL_BSDLCAEnableStatus_D/1
  LCDAL_BSDLCAEnableStatus_O/1 -> LCDAL_BSDLCAEnableStatus_st/2
  LCDAL_BSDLCAEnableStatus_sat/1 -> LCDAL_BSDLCAEnableStatus_st/1
  LCDAL_BSDLCAEnableStatus/1 -> LCDAL_BSDLCAEnableStatus_sat/1

== system VCU_CS75_10_9_SteeringTorque/长安CS75底盘程序，20ms一次/Output/Subsystem/TransmitMessages11/GW_LCDAL_2EA/LCDAL_BSDLCAStatus ==
  LCDAL_BSDLCAStatus : Inport
  Constant{1,3..8} (7 alike) : Constant  Value=0  OutDataTypeStr=uint8
  LCDAL_BSDLCAStatusRon : Rounding  Operator=round
  LCDAL_BSDLCAStatus_1sat : Saturate  UpperLimit=24  LowerLimit=0
  LCDAL_BSDLCAStatus_Convert : DataTypeConversion  OutDataTypeStr=uint8
  LCDAL_BSDLCAStatus_Convert1 : DataTypeConversion  OutDataTypeStr=uint32
  LCDAL_BSDLCAStatus_D : Product  Inputs=*/
  LCDAL_BSDLCAStatus_F : Constant  OutDataTypeStr=single
  LCDAL_BSDLCAStatus_L : simulink/Logic and Bit Operations/Bitwise Operator  logicop=AND  UseBitMask=on  BitMask=24  BitMaskRealWorld=Stored Integer
  LCDAL_BSDLCAStatus_O : Constant  Value=0  OutDataTypeStr=single
  LCDAL_BSDLCAStatus_S : ArithShift  BitShiftNumber=-3
  LCDAL_BSDLCAStatus_sat : Saturate  UpperLimit=3  LowerLimit=0
  LCDAL_BSDLCAStatus_st : Sum  Inputs=+-
  output1 : Outport
  output2 : Outport  Port=2
  output3 : Outport  Port=3
  output4 : Outport  Port=4
  output5 : Outport  Port=5
  output6 : Outport  Port=6
  output7 : Outport  Port=7
  output8 : Outport  Port=8
  wires:
  Constant8/1 -> output8/1
  Constant7/1 -> output7/1
  Constant6/1 -> output6/1
  Constant5/1 -> output5/1
  Constant4/1 -> output4/1
  Constant3/1 -> output3/1
  Constant1/1 -> output1/1
  LCDAL_BSDLCAStatus_Convert/1 -> output2/1
  LCDAL_BSDLCAStatus_L/1 -> LCDAL_BSDLCAStatus_Convert/1
  LCDAL_BSDLCAStatus_Convert1/1 -> LCDAL_BSDLCAStatus_L/1
  LCDAL_BSDLCAStatus_1sat/1 -> LCDAL_BSDLCAStatus_Convert1/1
  LCDAL_BSDLCAStatus_S/1 -> LCDAL_BSDLCAStatus_1sat/1
  LCDAL_BSDLCAStatusRon/1 -> LCDAL_BSDLCAStatus_S/1
  LCDAL_BSDLCAStatus_D/1 -> LCDAL_BSDLCAStatusRon/1
  LCDAL_BSDLCAStatus_F/1 -> LCDAL_BSDLCAStatus_D/2
  LCDAL_BSDLCAStatus_st/1 -> LCDAL_BSDLCAStatus_D/1
  LCDAL_BSDLCAStatus_O/1 -> LCDAL_BSDLCAStatus_st/2
  LCDAL_BSDLCAStatus_sat/1 -> LCDAL_BSDLCAStatus_st/1
  LCDAL_BSDLCAStatus/1 -> LCDAL_BSDLCAStatus_sat/1

== system VCU_CS75_10_9_SteeringTorque/长安CS75底盘程序，20ms一次/Output/Subsystem/TransmitMessages11/GW_LCDAL_2EA/LCDAL_CTAAlert ==
  LCDAL_CTAAlert : Inport
  Constant{2..8} (7 alike) : Constant  Value=0  OutDataTypeStr=uint8
  LCDAL_CTAAlertABS : Abs
  LCDAL_CTAAlertCS : ArithShift  BitShiftNumber=-2
  LCDAL_CTAAlertConS : Constant  OutDataTypeStr=single
  LCDAL_CTAAlertCosR : Constant  Value=0  OutDataTypeStr=uint8
  LCDAL_CTAAlertROP : RelationalOperator  Operator=<  OutDataTypeStr=boolean
  LCDAL_CTAAlertRon : Rounding  Operator=round
  LCDAL_CTAAlertSW : Switch  Criteria=u2 ~= 0
  LCDAL_CTAAlert_1sat : Saturate  UpperLimit=3  LowerLimit=0
  LCDAL_CTAAlert_Convert : DataTypeConversion  OutDataTypeStr=uint8
  LCDAL_CTAAlert_Convert1 : DataTypeConversion  OutDataTypeStr=uint32
  LCDAL_CTAAlert_D : Product  Inputs=*/
  LCDAL_CTAAlert_F : Constant  OutDataTypeStr=single
  LCDAL_CTAAlert_L : simulink/Logic and Bit Operations/Bitwise Operator  logicop=AND  UseBitMask=on  BitMask=3  BitMaskRealWorld=Stored Integer
  LCDAL_CTAAlert_O : Constant  Value=0  OutDataTypeStr=single
  LCDAL_CTAAlert_S : ArithShift
  LCDAL_CTAAlert_sat : Saturate  UpperLimit=3  LowerLimit=0
  LCDAL_CTAAlert_st : Sum  Inputs=+-
  LCDAL_CTAAlertsubcon : Sum  Inputs=+-
  output1 : Outport
  output2 : Outport  Port=2
  output3 : Outport  Port=3
  output4 : Outport  Port=4
  output5 : Outport  Port=5
  output6 : Outport  Port=6
  output7 : Outport  Port=7
  output8 : Outport  Port=8
  wires:
  Constant8/1 -> output8/1
  Constant7/1 -> output7/1
  Constant6/1 -> output6/1
  Constant5/1 -> output5/1
  Constant4/1 -> output4/1
  Constant3/1 -> output3/1
  Constant2/1 -> output2/1
  LCDAL_CTAAlert_Convert/1 -> output1/1
  LCDAL_CTAAlert_L/1 -> LCDAL_CTAAlert_Convert/1
  LCDAL_CTAAlert_Convert1/1 -> LCDAL_CTAAlert_L/1
  LCDAL_CTAAlert_1sat/1 -> LCDAL_CTAAlert_Convert1/1
  LCDAL_CTAAlert_S/1 -> LCDAL_CTAAlert_1sat/1
  LCDAL_CTAAlertSW/1 -> LCDAL_CTAAlert_S/1
  LCDAL_CTAAlertROP/1 -> LCDAL_CTAAlertSW/2
  LCDAL_CTAAlertsubcon/1 -> LCDAL_CTAAlertSW/1
  LCDAL_CTAAlertABS/1 -> LCDAL_CTAAlertsubcon/2
  LCDAL_CTAAlertCS/1 -> LCDAL_CTAAlertsubcon/1
  LCDAL_CTAAlertConS/1 -> LCDAL_CTAAlertCS/1
  LCDAL_CTAAlertCosR/1 -> LCDAL_CTAAlertROP/2
  LCDAL_CTAAlertRon/1 -> LCDAL_CTAAlertSW/3, LCDAL_CTAAlertABS/1, LCDAL_CTAAlertROP/1
  LCDAL_CTAAlert_D/1 -> LCDAL_CTAAlertRon/1
  LCDAL_CTAAlert_F/1 -> LCDAL_CTAAlert_D/2
  LCDAL_CTAAlert_st/1 -> LCDAL_CTAAlert_D/1
  LCDAL_CTAAlert_O/1 -> LCDAL_CTAAlert_st/2
  LCDAL_CTAAlert_sat/1 -> LCDAL_CTAAlert_st/1
  LCDAL_CTAAlert/1 -> LCDAL_CTAAlert_sat/1

== system VCU_CS75_10_9_SteeringTorque/长安CS75底盘程序，20ms一次/Output/Subsystem/TransmitMessages11/GW_LCDAL_2EA/LCDAL_CTAEnableStatus ==
  LCDAL_CTAEnableStatus : Inport
  Constant{1..3,5..8} (7 alike) : Constant  Value=0  OutDataTypeStr=uint8
  LCDAL_CTAEnableStatusRon : Rounding  Operator=round
  LCDAL_CTAEnableStatus_1sat : Saturate  UpperLimit=192  LowerLimit=0
  LCDAL_CTAEnableStatus_Convert : DataTypeConversion  OutDataTypeStr=uint8
  LCDAL_CTAEnableStatus_Convert1 : DataTypeConversion  OutDataTypeStr=uint32
  LCDAL_CTAEnableStatus_D : Product  Inputs=*/
  LCDAL_CTAEnableStatus_F : Constant  OutDataTypeStr=single
  LCDAL_CTAEnableStatus_L : simulink/Logic and Bit Operations/Bitwise Operator  logicop=AND  UseBitMask=on  BitMask=192  BitMaskRealWorld=Stored Integer
  LCDAL_CTAEnableStatus_O : Constant  Value=0  OutDataTypeStr=single
  LCDAL_CTAEnableStatus_S : ArithShift  BitShiftNumber=-6
  LCDAL_CTAEnableStatus_sat : Saturate  UpperLimit=3  LowerLimit=0
  LCDAL_CTAEnableStatus_st : Sum  Inputs=+-
  output1 : Outport
  output2 : Outport  Port=2
  output3 : Outport  Port=3
  output4 : Outport  Port=4
  output5 : Outport  Port=5
  output6 : Outport  Port=6
  output7 : Outport  Port=7
  output8 : Outport  Port=8
  wires:
  Constant8/1 -> output8/1
  Constant7/1 -> output7/1
  Constant6/1 -> output6/1
  Constant5/1 -> output5/1
  Constant3/1 -> output3/1
  Constant2/1 -> output2/1
  Constant1/1 -> output1/1
  LCDAL_CTAEnableStatus_Convert/1 -> output4/1
  LCDAL_CTAEnableStatus_L/1 -> LCDAL_CTAEnableStatus_Convert/1
  LCDAL_CTAEnableStatus_Convert1/1 -> LCDAL_CTAEnableStatus_L/1
  LCDAL_CTAEnableStatus_1sat/1 -> LCDAL_CTAEnableStatus_Convert1/1
  LCDAL_CTAEnableStatus_S/1 -> LCDAL_CTAEnableStatus_1sat/1
  LCDAL_CTAEnableStatusRon/1 -> LCDAL_CTAEnableStatus_S/1
  LCDAL_CTAEnableStatus_D/1 -> LCDAL_CTAEnableStatusRon/1
  LCDAL_CTAEnableStatus_F/1 -> LCDAL_CTAEnableStatus_D/2
  LCDAL_CTAEnableStatus_st/1 -> LCDAL_CTAEnableStatus_D/1
  LCDAL_CTAEnableStatus_O/1 -> LCDAL_CTAEnableStatus_st/2
  LCDAL_CTAEnableStatus_sat/1 -> LCDAL_CTAEnableStatus_st/1
  LCDAL_CTAEnableStatus/1 -> LCDAL_CTAEnableStatus_sat/1

== system VCU_CS75_10_9_SteeringTorque/长安CS75底盘程序，20ms一次/Output/Subsystem/TransmitMessages11/GW_LCDAL_2EA/LCDAL_CTAStatus ==
  LCDAL_CTAStatus : Inport
  Constant{1,3..8} (7 alike) : Constant  Value=0  OutDataTypeStr=uint8
  LCDAL_CTAStatusRon : Rounding  Operator=round
  LCDAL_CTAStatus_1sat : Saturate  UpperLimit=6  LowerLimit=0
  LCDAL_CTAStatus_Convert : DataTypeConversion  OutDataTypeStr=uint8
  LCDAL_CTAStatus_Convert1 : DataTypeConversion  OutDataTypeStr=uint32
  LCDAL_CTAStatus_D : Product  Inputs=*/
  LCDAL_CTAStatus_F : Constant  OutDataTypeStr=single
  LCDAL_CTAStatus_L : simulink/Logic and Bit Operations/Bitwise Operator  logicop=AND  UseBitMask=on  BitMask=6  BitMaskRealWorld=Stored Integer
  LCDAL_CTAStatus_O : Constant  Value=0  OutDataTypeStr=single
  LCDAL_CTAStatus_S : ArithShift  BitShiftNumber=-1
  LCDAL_CTAStatus_sat : Saturate  UpperLimit=3  LowerLimit=0
  LCDAL_CTAStatus_st : Sum  Inputs=+-
  output1 : Outport
  output2 : Outport  Port=2
  output3 : Outport  Port=3
  output4 : Outport  Port=4
  output5 : Outport  Port=5
  output6 : Outport  Port=6
  output7 : Outport  Port=7
  output8 : Outport  Port=8
  wires:
  Constant8/1 -> output8/1
  Constant7/1 -> output7/1
  Constant6/1 -> output6/1
  Constant5/1 -> output5/1
  Constant4/1 -> output4/1
  Constant3/1 -> output3/1
  Constant1/1 -> output1/1
  LCDAL_CTAStatus_Convert/1 -> output2/1
  LCDAL_CTAStatus_L/1 -> LCDAL_CTAStatus_Convert/1
  LCDAL_CTAStatus_Convert1/1 -> LCDAL_CTAStatus_L/1
  LCDAL_CTAStatus_1sat/1 -> LCDAL_CTAStatus_Convert1/1
  LCDAL_CTAStatus_S/1 -> LCDAL_CTAStatus_1sat/1
  LCDAL_CTAStatusRon/1 -> LCDAL_CTAStatus_S/1
  LCDAL_CTAStatus_D/1 -> LCDAL_CTAStatusRon/1
  LCDAL_CTAStatus_F/1 -> LCDAL_CTAStatus_D/2
  LCDAL_CTAStatus_st/1 -> LCDAL_CTAStatus_D/1
  LCDAL_CTAStatus_O/1 -> LCDAL_CTAStatus_st/2
  LCDAL_CTAStatus_sat/1 -> LCDAL_CTAStatus_st/1
  LCDAL_CTAStatus/1 -> LCDAL_CTAStatus_sat/1

== system VCU_CS75_10_9_SteeringTorque/长安CS75底盘程序，20ms一次/Output/Subsystem/TransmitMessages11/GW_LCDAL_2EA/LCDAL_LCATTCSettingStatus ==
  LCDAL_LCATTCSettingStatus : Inport
  Constant{1..4,6..8} (7 alike) : Constant  Value=0  OutDataTypeStr=uint8
  LCDAL_LCATTCSettingStatusABS : Abs
  LCDAL_LCATTCSettingStatusCS : ArithShift  BitShiftNumber=-2
  LCDAL_LCATTCSettingStatusConS : Constant  OutDataTypeStr=single
  LCDAL_LCATTCSettingStatusCosR : Constant  Value=0  OutDataTypeStr=uint8
  LCDAL_LCATTCSettingStatusROP : RelationalOperator  Operator=<  OutDataTypeStr=boolean
  LCDAL_LCATTCSettingStatusRon : Rounding  Operator=round
  LCDAL_LCATTCSettingStatusSW : Switch  Criteria=u2 ~= 0
  LCDAL_LCATTCSettingStatus_1sat : Saturate  UpperLimit=12  LowerLimit=0
  LCDAL_LCATTCSettingStatus_Convert : DataTypeConversion  OutDataTypeStr=uint8
  LCDAL_LCATTCSettingStatus_Convert1 : DataTypeConversion  OutDataTypeStr=uint32
  LCDAL_LCATTCSettingStatus_D : Product  Inputs=*/
  LCDAL_LCATTCSettingStatus_F : Constant  OutDataTypeStr=single
  LCDAL_LCATTCSettingStatus_L : simulink/Logic and Bit Operations/Bitwise Operator  logicop=AND  UseBitMask=on  BitMask=12  BitMaskRealWorld=Stored Integer
  LCDAL_LCATTCSettingStatus_O : Constant  Value=0  OutDataTypeStr=single
  LCDAL_LCATTCSettingStatus_S : ArithShift  BitShiftNumber=-2
  LCDAL_LCATTCSettingStatus_sat : Saturate  UpperLimit=3  LowerLimit=0
  LCDAL_LCATTCSettingStatus_st : Sum  Inputs=+-
  LCDAL_LCATTCSettingStatussubcon : Sum  Inputs=+-
  output1 : Outport
  output2 : Outport  Port=2
  output3 : Outport  Port=3
  output4 : Outport  Port=4
  output5 : Outport  Port=5
  output6 : Outport  Port=6
  output7 : Outport  Port=7
  output8 : Outport  Port=8
  wires:
  Constant8/1 -> output8/1
  Constant7/1 -> output7/1
  Constant6/1 -> output6/1
  Constant4/1 -> output4/1
  Constant3/1 -> output3/1
  Constant2/1 -> output2/1
  Constant1/1 -> output1/1
  LCDAL_LCATTCSettingStatus_Convert/1 -> output5/1
  LCDAL_LCATTCSettingStatus_L/1 -> LCDAL_LCATTCSettingStatus_Convert/1
  LCDAL_LCATTCSettingStatus_Convert1/1 -> LCDAL_LCATTCSettingStatus_L/1
  LCDAL_LCATTCSettingStatus_1sat/1 -> LCDAL_LCATTCSettingStatus_Convert1/1
  LCDAL_LCATTCSettingStatus_S/1 -> LCDAL_LCATTCSettingStatus_1sat/1
  LCDAL_LCATTCSettingStatusSW/1 -> LCDAL_LCATTCSettingStatus_S/1
  LCDAL_LCATTCSettingStatusROP/1 -> LCDAL_LCATTCSettingStatusSW/2
  LCDAL_LCATTCSettingStatussubcon/1 -> LCDAL_LCATTCSettingStatusSW/1
  LCDAL_LCATTCSettingStatusABS/1 -> LCDAL_LCATTCSettingStatussubcon/2
  LCDAL_LCATTCSettingStatusCS/1 -> LCDAL_LCATTCSettingStatussubcon/1
  LCDAL_LCATTCSettingStatusConS/1 -> LCDAL_LCATTCSettingStatusCS/1
  LCDAL_LCATTCSettingStatusCosR/1 -> LCDAL_LCATTCSettingStatusROP/2
  LCDAL_LCATTCSettingStatusRon/1 -> LCDAL_LCATTCSettingStatusSW/3, LCDAL_LCATTCSettingStatusABS/1, LCDAL_LCATTCSettingStatusROP/1
  LCDAL_LCATTCSettingStatus_D/1 -> LCDAL_LCATTCSettingStatusRon/1
  LCDAL_LCATTCSettingStatus_F/1 -> LCDAL_LCATTCSettingStatus_D/2
  LCDAL_LCATTCSettingStatus_st/1 -> LCDAL_LCATTCSettingStatus_D/1
  LCDAL_LCATTCSettingStatus_O/1 -> LCDAL_LCATTCSettingStatus_st/2
  LCDAL_LCATTCSettingStatus_sat/1 -> LCDAL_LCATTCSettingStatus_st/1
  LCDAL_LCATTCSettingStatus/1 -> LCDAL_LCATTCSettingStatus_sat/1

== system VCU_CS75_10_9_SteeringTorque/长安CS75底盘程序，20ms一次/Output/Subsystem/TransmitMessages11/GW_LCDAL_2EA/LCDAL_LockCtrlEnableStatus ==
  LCDAL_LockCtrlEnableStatus : Inport
  Constant{1..4,6..8} (7 alike) : Constant  Value=0  OutDataTypeStr=uint8
  LCDAL_LockCtrlEnableStatusABS : Abs
  LCDAL_LockCtrlEnableStatusCS : ArithShift  BitShiftNumber=-2
  LCDAL_LockCtrlEnableStatusConS : Constant  OutDataTypeStr=single
  LCDAL_LockCtrlEnableStatusCosR : Constant  Value=0  OutDataTypeStr=uint8
  LCDAL_LockCtrlEnableStatusROP : RelationalOperator  Operator=<  OutDataTypeStr=boolean
  LCDAL_LockCtrlEnableStatusRon : Rounding  Operator=round
  LCDAL_LockCtrlEnableStatusSW : Switch  Criteria=u2 ~= 0
  LCDAL_LockCtrlEnableStatus_1sat : Saturate  UpperLimit=48  LowerLimit=0
  LCDAL_LockCtrlEnableStatus_Convert : DataTypeConversion  OutDataTypeStr=uint8
  LCDAL_LockCtrlEnableStatus_Convert1 : DataTypeConversion  OutDataTypeStr=uint32
  LCDAL_LockCtrlEnableStatus_D : Product  Inputs=*/
  LCDAL_LockCtrlEnableStatus_F : Constant  OutDataTypeStr=single
  LCDAL_LockCtrlEnableStatus_L : simulink/Logic and Bit Operations/Bitwise Operator  logicop=AND  UseBitMask=on  BitMask=48  BitMaskRealWorld=Stored Integer
  LCDAL_LockCtrlEnableStatus_O : Constant  Value=0  OutDataTypeStr=single
  LCDAL_LockCtrlEnableStatus_S : ArithShift  BitShiftNumber=-4
  LCDAL_LockCtrlEnableStatus_sat : Saturate  UpperLimit=3  LowerLimit=0
  LCDAL_LockCtrlEnableStatus_st : Sum  Inputs=+-
  LCDAL_LockCtrlEnableStatussubcon : Sum  Inputs=+-
  output1 : Outport
  output2 : Outport  Port=2
  output3 : Outport  Port=3
  output4 : Outport  Port=4
  output5 : Outport  Port=5
  output6 : Outport  Port=6
  output7 : Outport  Port=7
  output8 : Outport  Port=8
  wires:
  Constant8/1 -> output8/1
  Constant7/1 -> output7/1
  Constant6/1 -> output6/1
  Constant4/1 -> output4/1
  Constant3/1 -> output3/1
  Constant2/1 -> output2/1
  Constant1/1 -> output1/1
  LCDAL_LockCtrlEnableStatus_Convert/1 -> output5/1
  LCDAL_LockCtrlEnableStatus_L/1 -> LCDAL_LockCtrlEnableStatus_Convert/1
  LCDAL_LockCtrlEnableStatus_Convert1/1 -> LCDAL_LockCtrlEnableStatus_L/1
  LCDAL_LockCtrlEnableStatus_1sat/1 -> LCDAL_LockCtrlEnableStatus_Convert1/1
  LCDAL_LockCtrlEnableStatus_S/1 -> LCDAL_LockCtrlEnableStatus_1sat/1
  LCDAL_LockCtrlEnableStatusSW/1 -> LCDAL_LockCtrlEnableStatus_S/1
  LCDAL_LockCtrlEnableStatusROP/1 -> LCDAL_LockCtrlEnableStatusSW/2
  LCDAL_LockCtrlEnableStatussubcon/1 -> LCDAL_LockCtrlEnableStatusSW/1
  LCDAL_LockCtrlEnableStatusABS/1 -> LCDAL_LockCtrlEnableStatussubcon/2
  LCDAL_LockCtrlEnableStatusCS/1 -> LCDAL_LockCtrlEnableStatussubcon/1
  LCDAL_LockCtrlEnableStatusConS/1 -> LCDAL_LockCtrlEnableStatusCS/1
  LCDAL_LockCtrlEnableStatusCosR/1 -> LCDAL_LockCtrlEnableStatusROP/2
  LCDAL_LockCtrlEnableStatusRon/1 -> LCDAL_LockCtrlEnableStatusSW/3, LCDAL_LockCtrlEnableStatusABS/1, LCDAL_LockCtrlEnableStatusROP/1
  LCDAL_LockCtrlEnableStatus_D/1 -> LCDAL_LockCtrlEnableStatusRon/1
  LCDAL_LockCtrlEnableStatus_F/1 -> LCDAL_LockCtrlEnableStatus_D/2
  LCDAL_LockCtrlEnableStatus_st/1 -> LCDAL_LockCtrlEnableStatus_D/1
  LCDAL_LockCtrlEnableStatus_O/1 -> LCDAL_LockCtrlEnableStatus_st/2
  LCDAL_LockCtrlEnableStatus_sat/1 -> LCDAL_LockCtrlEnableStatus_st/1
  LCDAL_LockCtrlEnableStatus/1 -> LCDAL_LockCtrlEnableStatus_sat/1
